simulink model "untitled"  (R2021b)
settings: Solver=ode45  StartTime=0.0  StopTime=3000  FixedStep=0.0001  RelTol=1e-3
settings Model: Creator=Asus  LastModifiedBy=Asus

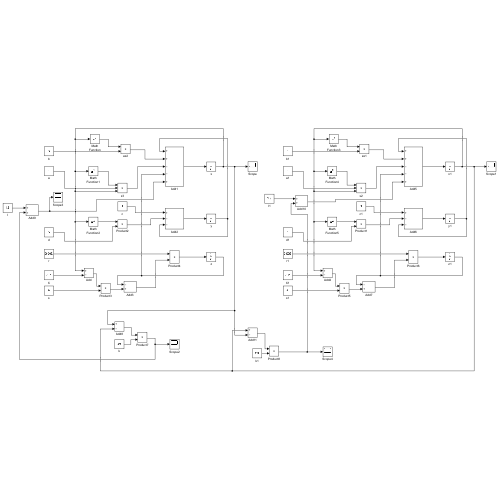
[thumbnail: Simulink's stored preview of the top-level diagram]
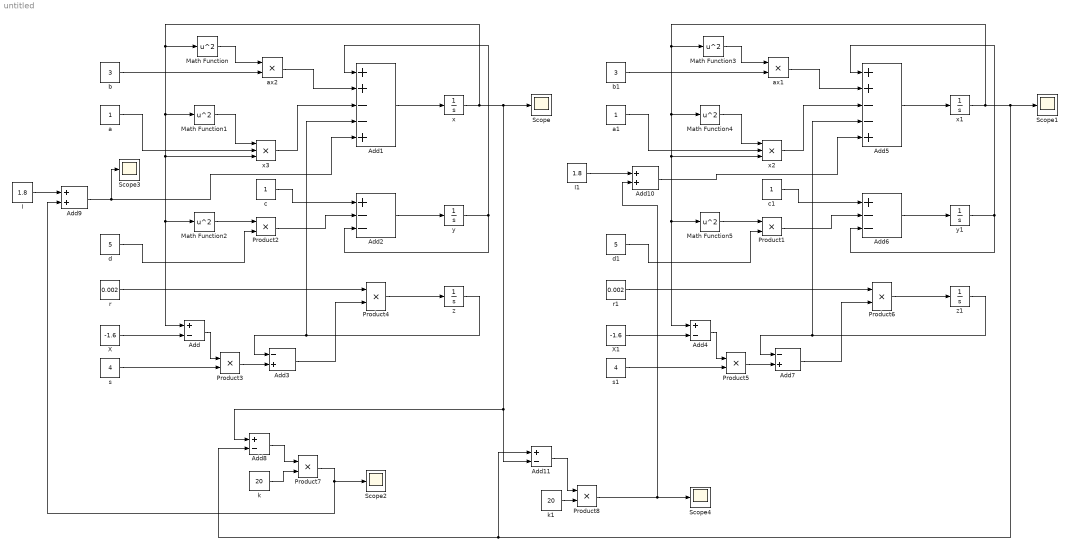
== system untitled ==
  Add{,4,8,11} (4 alike) : Sum  Inputs=+-
  Add1 : Sum  Inputs=++--+
  Add10 : Sum
  Add2 : Sum  Inputs=+--
  Add3 : Sum  Inputs=-+
  Add5 : Sum  Inputs=++--+
  Add6 : Sum  Inputs=+--
  Add7 : Sum  Inputs=-+
  Add9 : Sum
  I : Constant  Value=1.8
  I1 : Constant  Value=1.8
  Math Function{,1..5} (6 alike) : Math  Operator=square  SaturateOnIntegerOverflow=on
  Product{1..8} (8 alike) : Product
  Scope{,1..4} (5 alike) : Scope
  X : Constant  Value=-1.6
  X1 : Constant  Value=-1.6
  a : Constant
  a1 : Constant
  ax1 : Product
  ax2 : Product
  b : Constant  Value=3
  b1 : Constant  Value=3
  c : Constant
  c1 : Constant
  d : Constant  Value=5
  d1 : Constant  Value=5
  k : Constant  Value=20
  k1 : Constant  Value=20
  r : Constant  Value=0.002
  r1 : Constant  Value=0.002
  s : Constant  Value=4
  s1 : Constant  Value=4
  x : Integrator
  x1 : Integrator
  x2 : Product  Inputs=3
  x3 : Product  Inputs=3
  y : Integrator
  y1 : Integrator
  z : Integrator
  z1 : Integrator
  wires:
  Math Function1/1 -> x3/1
  Math Function/1 -> ax2/1
  Math Function2/1 -> Product2/1
  Add/1 -> Product3/1
  ax2/1 -> Add1/2
  x3/1 -> Add1/3
  c/1 -> Add2/1
  Product2/1 -> Add2/2
  Add1/1 -> x/1
  Add2/1 -> y/1
  x/1 -> Add11/2, Add8/1, Scope/1, Add/1, Math Function2/1, x3/3, Math Function1/1, Math Function/1
  y/1 -> Add2/3, Add1/1
  z/1 -> Add3/1, Add1/4
  d/1 -> Product2/2
  X/1 -> Add/2
  s/1 -> Product3/2
  Product3/1 -> Add3/2
  Add3/1 -> Product4/2
  r/1 -> Product4/1
  Product4/1 -> z/1
  a/1 -> x3/2
  b/1 -> ax2/2
  Add6/1 -> y1/1
  Product1/1 -> Add6/2
  x2/1 -> Add5/3
  y1/1 -> Add6/3, Add5/1
  Math Function5/1 -> Product1/1
  Add5/1 -> x1/1
  Product5/1 -> Add7/2
  r1/1 -> Product6/1
  Product6/1 -> z1/1
  b1/1 -> ax1/2
  d1/1 -> Product1/2
  Add4/1 -> Product5/1
  Math Function4/1 -> x2/1
  Add7/1 -> Product6/2
  X1/1 -> Add4/2
  c1/1 -> Add6/1
  ax1/1 -> Add5/2
  a1/1 -> x2/2
  z1/1 -> Add7/1, Add5/4
  s1/1 -> Product5/2
  Math Function3/1 -> ax1/1
  x1/1 -> Add11/1, Add8/2, Scope1/1, Add4/1, Math Function5/1, x2/3, Math Function4/1, Math Function3/1
  Add8/1 -> Product7/1
  k/1 -> Product7/2
  I/1 -> Add9/1
  Product7/1 -> Add9/2, Scope2/1
  Add9/1 -> Scope3/1, Add1/5
  k1/1 -> Product8/2
  Add10/1 -> Add5/5
  I1/1 -> Add10/1
  Product8/1 -> Add10/2, Scope4/1
  Add11/1 -> Product8/1
